simulink model "pltl_identities"  (R2014a)
settings: Solver=FixedStepDiscrete  StartTime=0.0  StopTime=inf  RelTol=1e-3
libraries: patterns_library x12, sldvlib x6
settings Model: Creator=lgwagner  LastModifiedBy=lgwagner

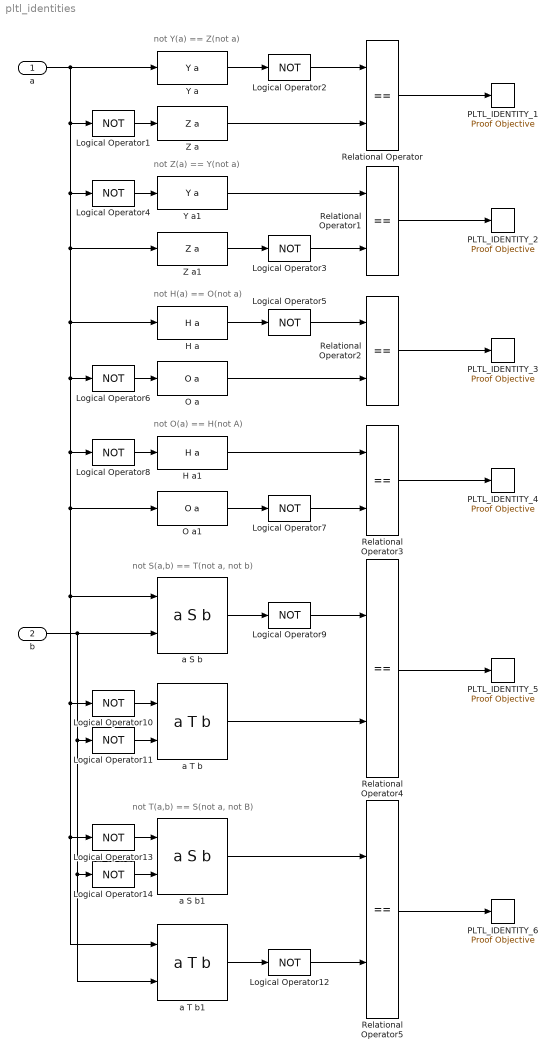
== system pltl_identities ==
  note: not Y(a) == Z(not a)
  note: not Z(a) == Y(not a)
  note: not H(a) == O(not a)
  note: not O(a) == H(not A)
  note: not S(a,b) == T(not a, not b)
  note: not T(a,b) == S(not a, not B)
  a : Inport  OutDataTypeStr=boolean
  b : Inport  Port=2  OutDataTypeStr=boolean
  H a : patterns_library/H a
  H a1 : patterns_library/H a
  Logical Operator{1..14} (14 alike) : Logic  Operator=NOT  AllPortsSameDT=off  OutDataTypeStr=boolean
  O a : patterns_library/O a
  O a1 : patterns_library/O a
  PLTL_IDENTITY_{1..6} (6 alike) : sldvlib/Objectives and Constraints/Proof Objective  enabled=on  customAVTBlockType=Proof Objective  intervals=true  dispValues=on  outEnabled=off  enableStopSim=off
      settings: AttributesFormatString=%<intervals>
  Relational Operator{,1..5} (6 alike) : RelationalOperator  Operator===  OutDataTypeStr=boolean
  Y a : patterns_library/Y a
  Y a1 : patterns_library/Y a
  Z a : patterns_library/Z a
  Z a1 : patterns_library/Z a
  a S b : patterns_library/a S b
  a S b1 : patterns_library/a S b
  a T b : patterns_library/a T b
  a T b1 : patterns_library/a T b
  wires:
  a/1 -> Logical Operator1/1, Logical Operator6/1, Logical Operator10/1, a T b1/1, Logical Operator13/1, a S b/1, O a1/1, Logical Operator8/1, H a/1, Z a1/1, Logical Operator4/1, Y a/1
  Y a/1 -> Logical Operator2/1
  Relational Operator/1 -> PLTL_IDENTITY_1/1
  Z a/1 -> Relational Operator/2
  Logical Operator2/1 -> Relational Operator/1
  Logical Operator1/1 -> Z a/1
  Relational Operator1/1 -> PLTL_IDENTITY_2/1
  Z a1/1 -> Logical Operator3/1
  Y a1/1 -> Relational Operator1/1
  Logical Operator3/1 -> Relational Operator1/2
  Logical Operator4/1 -> Y a1/1
  H a/1 -> Logical Operator5/1
  O a/1 -> Relational Operator2/2
  Logical Operator5/1 -> Relational Operator2/1
  Logical Operator6/1 -> O a/1
  Relational Operator2/1 -> PLTL_IDENTITY_3/1
  O a1/1 -> Logical Operator7/1
  H a1/1 -> Relational Operator3/1
  Relational Operator3/1 -> PLTL_IDENTITY_4/1
  Logical Operator7/1 -> Relational Operator3/2
  Logical Operator8/1 -> H a1/1
  a T b/1 -> Relational Operator4/2
  a S b/1 -> Logical Operator9/1
  b/1 -> a T b1/2, Logical Operator14/1, Logical Operator11/1, a S b/2
  Relational Operator4/1 -> PLTL_IDENTITY_5/1
  a T b1/1 -> Logical Operator12/1
  a S b1/1 -> Relational Operator5/1
  Relational Operator5/1 -> PLTL_IDENTITY_6/1
  Logical Operator9/1 -> Relational Operator4/1
  Logical Operator10/1 -> a T b/1
  Logical Operator11/1 -> a T b/2
  Logical Operator12/1 -> Relational Operator5/2
  Logical Operator13/1 -> a S b1/1
  Logical Operator14/1 -> a S b1/2
